simulink model "PVTOL_PseudoSMC"  (R2026b)
settings Model: Creator=nestorhernandezcastellanos  LastModifiedBy=nestorhernandezcastellanos

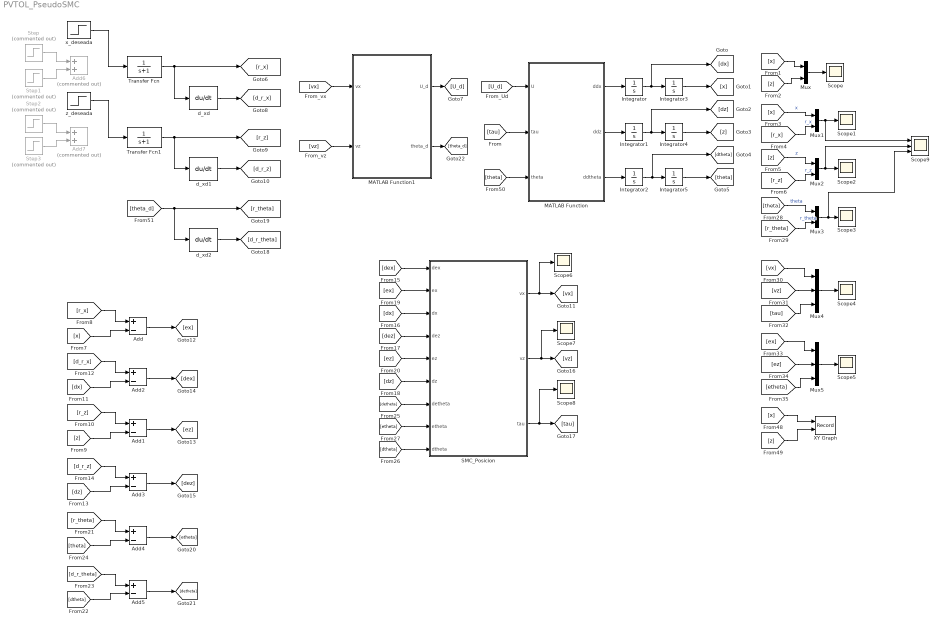
== system PVTOL_PseudoSMC ==
  Add{,1..5} (6 alike) : Sum  Inputs=+-
  Add6 : Sum  Commented=on
  Add7 : Sum  Commented=on
  Integrator{,1..5} (6 alike) : Integrator
  MATLAB Function : MATLAB Function  TreatAsAtomicUnit=on
  MATLAB Function1 : MATLAB Function  TreatAsAtomicUnit=on
  Mux{,1..3} (4 alike) : Mux  Inputs=2
  Mux4 : Mux  Inputs=3
  Mux5 : Mux  Inputs=3
  SMC_Posicion : MATLAB Function  TreatAsAtomicUnit=on
  Scope{,1..8} (9 alike) : Scope
      Scope settings: ActiveDisplayYMinimum=0.024738728132078558  ActiveDisplayYMaximum=5.5528067767038412
      Scope1 settings: ActiveDisplayYMinimum=-0.62499999649831228  ActiveDisplayYMaximum=5.6249999684848113
      Scope2 settings: ActiveDisplayYMinimum=-0.62499999649831228  ActiveDisplayYMaximum=5.6249999684848113  DataLoggingVariableName=ScopeData2
      Scope3 settings: ActiveDisplayYMinimum=-2.37928301075874  ActiveDisplayYMaximum=21.413547096828665  DataLoggingVariableName=ScopeData3
      Scope4 settings: ActiveDisplayYMinimum=-7.3436048207987019  ActiveDisplayYMaximum=6.2474960105062456  DataLoggingVariableName=ScopeData4
      Scope5 settings: ActiveDisplayYMinimum=-1.0091994284829338  ActiveDisplayYMaximum=3.4185330784233448  DataLoggingVariableName=ScopeData5
      Scope6 settings: ActiveDisplayYMinimum=-21.515643312433614  ActiveDisplayYMaximum=3.2981489512032809  DataLoggingVariableName=ScopeData6
      Scope7 settings: ActiveDisplayYMinimum=-21.515643312433614  ActiveDisplayYMaximum=3.2981489512032809  DataLoggingVariableName=ScopeData7
      Scope8 settings: ActiveDisplayYMinimum=-21.515643312433614  ActiveDisplayYMaximum=3.2981489512032809  DataLoggingVariableName=ScopeData8
  Scope9 : Scope  NumInputPorts=3
      settings: ActiveDisplayYMinimum=-0.63188691193482271  ActiveDisplayYMaximum=5.6869822074134051  DataLoggingVariableName=ScopeData9
  Step : Step  Commented=on  FinalValue=3  SampleTime=0
  Step1 : Step  Commented=on  Time=15  FinalValue=7  SampleTime=0
  Step2 : Step  Commented=on  FinalValue=3  SampleTime=0
  Step3 : Step  Commented=on  Time=15  FinalValue=7  SampleTime=0
  Transfer Fcn : TransferFcn  Denominator=[1 1]
  Transfer Fcn1 : TransferFcn  Denominator=[1 1]
  XY Graph : Record  NumPorts=2.0  FileSettingsInternal="{\"entries\":[{\"content\":{\"excelSettings\":{\"content\":{},\"type\":\"Streamout.ExcelSettings\"},\"parquetSettings\":{\"content\":{},\"type\":\"Streamout.ParquetSettings\"}},\"type\":\"Streamout.FileSettingStorage\",\"uuid\":\"\"}],\"packageUris\":[\"http:\\/\\/schema.mathworks.com\\/mf0\\/streamout_blocks\\/R2020a\"],\"version\":\"1.0\"}"  FrameSettings=[0, 0]  Layout=[1 1]  SignalsInternal="{\"entries\":[{\"content\":{\"signals\":[{\"content\":{\"blockPath\":[],\"dimensions\":[1],\"domain\":\"\",\"lineColor\":\"#a2142f\",\"plots\":[ 1 ],\"port\":1,\"sid\":[\"\"],\"signalID\":1,\"signalName\":\"From48\"},\"type\":\"RecordBlkView.Signal\",\"uuid\":\"\"},{\"content\":{\"blockPath\":[],\"dimensions\":[1],\"domain\":\"\",\"lineColor\":\"#139fff\",\"plots\":[ 1 ],\"port\":2,\"sid\":[\"\"],\"signalID\":2,\"signalName\":\"From49\"},\"type\":\"RecordBlkView.Signal\",\"uuid\":\"\"}]},\"type\":\"RecordBlkView.InputSignals\",\"uuid\":\"\"}],\"packageUris\":[\"http:\\/\\/schema.mathworks.com\\/mf0\\/streamout_blocks\\/R2020a\"],\"version\":\"1.0\"}"  VisualizationBindings="{\"xyplotplugin\":{\"info\":[{\"series\":[{\"bindingParametersList\":[{\"parameter\":\"X-Axis\",\"signalID\":1,\"signalName\":\"From48\"},{\"parameter\":\"Y-Axis\",\"signalID\":2,\"signalName\":\"From49\"}],\"seriesID\":0}],\"subplotID\":1}]}}"  CompatibilityTag=XY
  d_xd : Derivative
  d_xd1 : Derivative
  d_xd2 : Derivative
  x_deseada : Step  FinalValue=5  SampleTime=0
  z_deseada : Step  FinalValue=5  SampleTime=0
  wires:
  Mux/1 -> Scope/1
  [z] -> Mux/2
  [x] -> Mux/1
  [x] -> Mux1/1  "x"
  [r_x] -> Mux1/2  "r_x"
  [r_z] -> Mux2/2  "r_z"
  [z] -> Mux2/1  "z"
  [r_x] -> Add/1
  [x] -> Add/2
  Add/1 -> [ex]
  Add1/1 -> [ez]
  [z] -> Add1/2
  [r_z] -> Add1/1
  Add2/1 -> [dex]
  [dx] -> Add2/2
  [d_r_x] -> Add2/1
  [d_r_z] -> Add3/1
  [dz] -> Add3/2
  Add3/1 -> [dez]
  SMC_Posicion/1(vx) -> Scope6/1, [vx]
  SMC_Posicion/2(vz) -> Scope7/1, [vz]
  SMC_Posicion/3(tau) -> Scope8/1, [tau]
  [dex] -> SMC_Posicion/1(dex)
  [dx] -> SMC_Posicion/3(dx)
  [dez] -> SMC_Posicion/4(dez)
  [dz] -> SMC_Posicion/6(dz)
  [ex] -> SMC_Posicion/2(ex)
  [ez] -> SMC_Posicion/5(ez)
  Add5/1 -> [detheta]
  [dtheta] -> Add5/2
  [d_r_theta] -> Add5/1
  [r_theta] -> Add4/1
  [theta] -> Add4/2
  Add4/1 -> [etheta]
  [detheta] -> SMC_Posicion/7(detheta)
  [etheta] -> SMC_Posicion/8(etheta)
  [dtheta] -> SMC_Posicion/9(dtheta)
  [theta] -> Mux3/1  "theta"
  [r_theta] -> Mux3/2  "r_theta"
  Mux4/1 -> Scope4/1
  [vz] -> Mux4/2
  [vx] -> Mux4/1
  [tau] -> Mux4/3
  [etheta] -> Mux5/3
  [ex] -> Mux5/1
  [ez] -> Mux5/2
  Mux5/1 -> Scope5/1
  Integrator5/1 -> [theta]
  [theta_d] -> [r_theta], d_xd2/1
  Integrator3/1 -> [x]
  [tau] -> MATLAB Function/2(tau)
  x_deseada/1 -> Transfer Fcn/1
  [theta] -> MATLAB Function/3(theta)
  [vx] -> MATLAB Function1/1(vx)
  MATLAB Function1/1(U_d) -> [U_d]
  d_xd2/1 -> [d_r_theta]
  Transfer Fcn1/1 -> d_xd1/1, [r_z]
  Step3/1 -> Add7/2
  MATLAB Function/1(ddx) -> Integrator/1
  Step/1 -> Add6/1
  Step2/1 -> Add7/1
  Integrator1/1 -> [dz], Integrator4/1
  Integrator4/1 -> [z]
  MATLAB Function/3(ddtheta) -> Integrator2/1
  Integrator/1 -> [dx], Integrator3/1
  MATLAB Function1/2(theta_d) -> [theta_d]
  [U_d] -> MATLAB Function/1(U)
  MATLAB Function/2(ddz) -> Integrator1/1
  [vz] -> MATLAB Function1/2(vz)
  d_xd1/1 -> [d_r_z]
  Step1/1 -> Add6/2
  Integrator2/1 -> [dtheta], Integrator5/1
  d_xd/1 -> [d_r_x]
  Transfer Fcn/1 -> [r_x], d_xd/1
  z_deseada/1 -> Transfer Fcn1/1
  [x] -> XY Graph/1
  [z] -> XY Graph/2
  Mux1/1 -> Scope9/1, Scope1/1
  Mux3/1 -> Scope9/3, Scope3/1
  Mux2/1 -> Scope9/2, Scope2/1

== matlab function PVTOL_PseudoSMC/MATLAB Function1 ==
  data: vx input; U_d output; vz input; theta_d output
function [U_d,theta_d] = linealizacion(vx,vz)

g = 9.81;                                  
U_d = sqrt(vx^2 + (vz+g)^2);                 
theta_d = atan2(-vx,vz+g);

== matlab function PVTOL_PseudoSMC/MATLAB Function ==
  data: U input; ddx output; tau input; theta input; ddz output; ddtheta output
function [ddx,ddz,ddtheta] = planta(U,tau,theta)

g = 9.81;                                       

ddx = -U*sin(theta);                            
ddz = U*cos(theta)-g;                           
ddtheta = tau;

== matlab function PVTOL_PseudoSMC/SMC_Posicion ==
  data: dex input; ex input; dx input; vx output; dez input; ez input; dz input; vz output; tau output; detheta input; etheta input; dtheta input
function [vx, vz, tau] = controlador(dex, ex, dx, dez, ez, dz, detheta, etheta, dtheta)

% Parámetros de las superficies de deslizamiento
mx = 2;
mz = 2;
mtheta = 2;

% Ganancias del controlador
Kx = 6;
Kz = 4;
Ktheta = 8;

% Amplitudes de las funciones de saturación
Lx = 0.5;
Lz = 0.5;
Ltheta = 0.5;

% Parámetros de pendiente
eta_x = 0.20;
eta_z = 0.20;
eta_theta = 0.10;

% Superficies de pseudo modo deslizante
sigma_x = dex + mx*ex;
sigma_z = dez + mz*ez;
sigma_theta = detheta + mtheta*etheta;

% Funciones de saturación
sat_x = max(-Lx, min(Lx, sigma_x/eta_x));
sat_z = max(-Lz, min(Lz, sigma_z/eta_z));
sat_theta = max(-Ltheta, min(Ltheta, sigma_theta/eta_theta));

% Entradas virtuales
vx = -mx*dx + Kx*sat_x;
vz = -mz*dz + Kz*sat_z;

% Control de actitud
tau = -mtheta*dtheta + Ktheta*sat_theta;
